simulink model "System_generator_top"  (R2025b)
settings: Solver=FixedStepAuto  StartTime=0.0  StopTime=10560000  FixedStep=1  RelTol=1e-3
InitFcn:
  | % 1. Dynamically find the exact folder where your .slx model file is saved
  | model_full_path = get_param(bdroot, 'FileName');
  | [project_dir, ~, ~] = fileparts(model_full_path);
  | input_file_path = fullfile(project_dir, 'input_video.txt');
  | 
  | % 2. Load the file directly from that project folder
  | if exist(input_file_path, 'file')
  |     fileID = fopen(input_file_path, 'r');
  |     file_contents = textscan(fileID, '%s');
  |     fclose(fileID);
  |     try
  |         raw_pixels = hex2dec(file_contents{1});
  |     catch
  |         raw_pixels = readmatrix(input_file_path);
  |         raw_pixels = raw_pixels(~isnan(raw_pixels));
  |     end
  |     total_cycles = length(raw_pixels);
  |     assignin('base', 'input_stream', [(0:total_cycles-1)', raw_pixels]);
  | 
  |     % --- THE AUTOMATION LEVEL-UP ---
  |     % Force the Simulink model stop time box to match the exact size of the video file
  |     set_param(bdroot, 'StopTime', num2str(total_cycles));
  |     fprintf('--> Automation Success: Simulink StopTime auto-set to %d to match total text pixels.\n', total_cycles);
  |     % ---------------------------------
  | else
  |     warndlg(['Warning: input_video.txt was not found in your project folder: ', project_dir]);
  | end
StopFcn:
  | try
  |     % 1. Find exactly where input_video.txt is stored
  |     input_file_full_path = which('input_video.txt');
  |     if ~isempty(input_file_full_path)
  |         [target_dir, ~, ~] = fileparts(input_file_full_path);
  |     else
  |         model_full_path = get_param(bdroot, 'FileName');
  |         [target_dir, ~, ~] = fileparts(model_full_path);
  |     end
  | 
  |     % ==========================================================
  |     % 2. STREAM EDGE PIXELS TO "output_edges.txt"
  |     % ==========================================================
  |     if exist('out', 'var') && (isprop(out, 'output_pixels') || isfield(out, 'output_pixels'))
  |         raw_output = out.output_pixels;
  |     else
  |         error('No output pixel variable found in the workspace.');
  |     end
  | 
  |     if isa(raw_output, 'Simulink.SimulationData.Signal')
  |         processed_data = raw_output.Values.Data;
  |     elseif isa(raw_output, 'timeseries')
  |         processed_data = raw_output.Data;
  |     else
  |         processed_data = raw_output;
  |     end
  | 
  |     processed_data = squeeze(double(processed_data));
  | 
  |     final_output_path = fullfile(target_dir, 'output_edges.txt');
  |     fileID = fopen(final_output_path, 'w');
  |     fprintf(fileID, '%02x\n', uint8(processed_data));
  |     fclose(fileID);
  |     fprintf('--> Automation Success: "output_edges.txt" saved.\n');
  | 
  |     % ==========================================================
  |     % 3. STREAM COORDINATES TO "box_coordinates.txt"
  |     % ==========================================================
  |     if isprop(out, 'box_min_x') || isfield(out, 'box_min_x')
  |         % Robust extraction for both Signal structures and raw timeseries classes
  |         if isa(out.box_min_x, 'Simulink.SimulationData.Signal')
  |             bx = out.box_min_x.Values.Data; Bx = out.box_max_x.Values.Data;
  |             by = out.box_min_y.Values.Data; By = out.box_max_y.Values.Data;
  |         elseif isa(out.box_min_x, 'timeseries')
  |             bx = out.box_min_x.Data; Bx = out.box_max_x.Data;
  |             by = out.box_min_y.Data; By = out.box_max_y.Data;
  |         else
  |             bx = out.box_min_x; Bx = out.box_max_x;
  |             by = out.box_min_y; By = out.box_max_y;
  |         end
  | 
  |         bx = squeeze(double(bx)); Bx = squeeze(double(Bx));
  |         by = squeeze(double(by)); By = squeeze(double(By));
  | 
  |         coords_matrix = [bx, Bx, by, By];
  | 
  |         final_coords_path = fullfile(target_dir, 'box_coordinates.txt');
  |         fileID_coords = fopen(final_coords_path, 'w');
  |         fprintf(fileID_coords, '%d %d %d %d\n', coords_matrix');
  |         fclose(fileID_coords);
  |         fprintf('--> Automation Success: "box_coordinates.txt" saved directly to your folder.\n');
  |     else
  |         warning('Coordinates missing from output structure! Check your To Workspace block names.');
  |     end
  | 
  | catch ME
  |     warning('Automation Failed: %s', ME.message);
  | end
undefined symbols (not defined in the file): gray, Subsystem, System_generator_top_exp_donot_USE, xc7z010clg400
libraries: hdlBasic x14, vmcUtilities x1
settings Model: Creator=Mayur  LastModifiedBy=Mayur

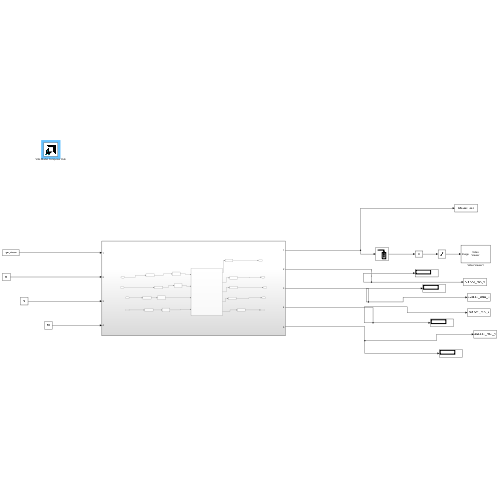
[thumbnail: Simulink's stored preview of the top-level diagram]
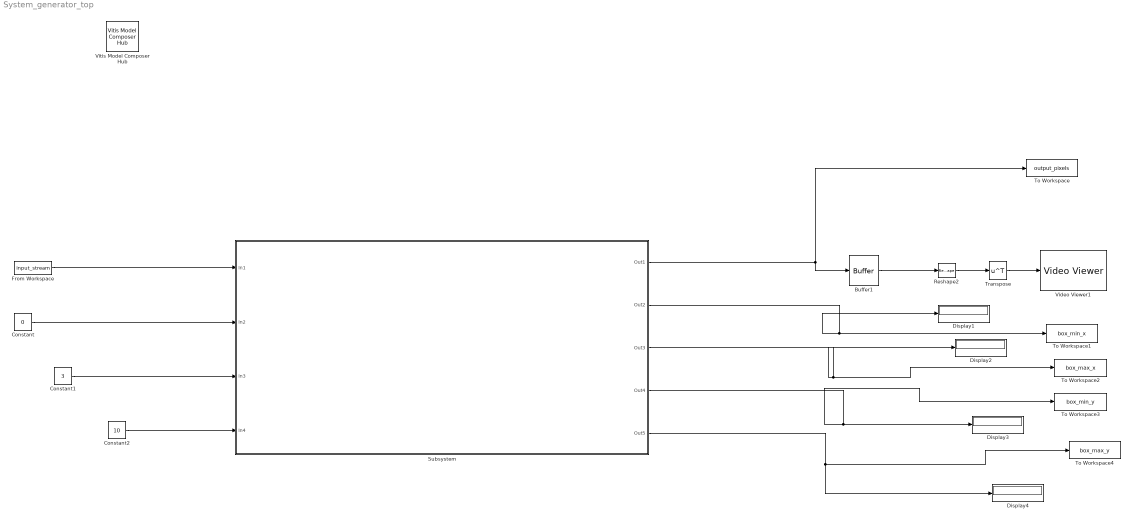
== system System_generator_top ==
  Buffer1 : Buffer  N=19200  OutputFrames=off
  Constant : Constant  Value=0  SampleTime=1  LockScale=on
  Constant1 : Constant  Value=3  SampleTime=1
  Constant2 : Constant  Value=10
  Display{1..4} (4 alike) : Display
  From Workspace : FromWorkspace  VariableName=input_stream  SampleTime=1  Interpolate=off  OutputAfterFinalValue=Holding final value
  Reshape2 : Reshape  OutputDimensionality=Customize  OutputDimensions=[160,120]
  Subsystem : Subsystem
  To Workspace : ToWorkspace  VariableName=output_pixels  SaveFormat=Timeseries  SampleTime=-1
  To Workspace1 : ToWorkspace  VariableName=box_min_x  SaveFormat=Timeseries  SampleTime=-1
  To Workspace2 : ToWorkspace  VariableName=box_max_x  SaveFormat=Timeseries  SampleTime=-1
  To Workspace3 : ToWorkspace  VariableName=box_min_y  SaveFormat=Timeseries  SampleTime=-1
  To Workspace4 : ToWorkspace  VariableName=box_max_y  SaveFormat=Timeseries  SampleTime=-1
  Transpose : Math  Operator=transpose
  Video Viewer1 : VideoViewer  colormapValue=gray(256)  FigPos=[893 880.666666666667 660 613]
  Vitis Model Composer Hub : vmcUtilities/Vitis Model Composer Hub  Tag=genX  CodeGeneration=off  SubsystemName=Subsystem  BlockHierPath=System_generator_top_exp_donot_USE/Subsystem  CompilationType=HDLCompilation  SubsystemType=HDLNode  ExportTypeV2=HDL Netlist  StartColumn=1  NumberOfColumns=1  TargetDirectory=C:/Users/Mayur/AppData/Roaming/Xilinx/Sysgen  exportDesign=on  analyzeDesign=off  validateDesignOnHw=off  ExportType=AI Engines  IpVendor=xilinx.com  IpLibrary=hls  IpVersion=1.0  IpHWLanguage=Verilog  AieCompilerOptions={}  AieSimulatorOptions={}  CreateTestbench=off  TestbenchStackSize=10  RunRtlSim=off  RunCSim=off  RunAieSim=off  AieSimTimeout=50000  RunAieSimProfiling=off  LaunchVitisAnalyzer=off  PlotOutput=off  RunX86Sim=off  X86SimTimeout=10  GenHwImage=off  GenLibadfXo=on  GenHwValidationCode=off  PlatformType=Not Specified  HwSystemType=Baremetal  HwValidationTarget=hw  ProjDevice=xc7z010clg400-1  ProjDevicePart=xc7z010clg400-1  AIEType=None  SamplePeriod=-1  ClockFrequency=200  DataPathParallelism=1  xilinxfamily=zynq  part=xc7z010  speed=-1  package=clg400  directory=./netlist\ip\Subsystem\src  testbench=off  incr_netlist=off  synthesis_tool=Vivado  clock_wrapper=Clock Enables  dbl_ovrd=According to Block Masks  dcm_input_clock_period=10  sysclk_period=10  simulink_period=1  eval_field=0  IPInfoJsonString="{\"DUTSubsystemName\":\"Subsystem\",\"HDLSubsystem\":{\"SubsystemName\":\"Subsystem\",\"IPName\":\"Subsystem\",\"IPLibrary\":\"VMC\",\"IPVendor\":\"User Company\",\"IPVersion\":\"1.0\",\"TargetDirectory\":\"C:/Users/Mayur/AppData/Roaming/Xilinx/Sysgen\",\"SubsystemDir\":\"C:/Users/Mayur/AppData/Roaming/Xilinx/Sysgen\\\\ip\\\\Subsystem\",\"FreqHz\":\"100000000\"},\"SubsystemTag\":\"HDLNode\"}"  LogFileName=C:\Users\Mayur\AppData\Roaming\Xilinx\Sysgen\model_composer.log  NThreads=4  IPConfigFile=C:\Users\Mayur\AppData\Local\Temp\vmctmp-14156349143152141850\System_generator_top_exp_donot_USE_ipconfig.json
  wires:
  Buffer1/1 -> Reshape2/1
  Reshape2/1 -> Transpose/1
  Transpose/1 -> Video Viewer1/1
  Subsystem/5(Out5) -> Display4/1, To Workspace4/1
  Subsystem/4(Out4) -> To Workspace3/1, Display3/1
  Subsystem/1(Out1) -> To Workspace/1, Buffer1/1
  Subsystem/2(Out2) -> Display1/1, To Workspace1/1
  Subsystem/3(Out3) -> To Workspace2/1, Display2/1
  From Workspace/1 -> Subsystem/1(In1)
  Constant/1 -> Subsystem/2(In2)
  Constant1/1 -> Subsystem/3(In3)
  Constant2/1 -> Subsystem/4(In4)

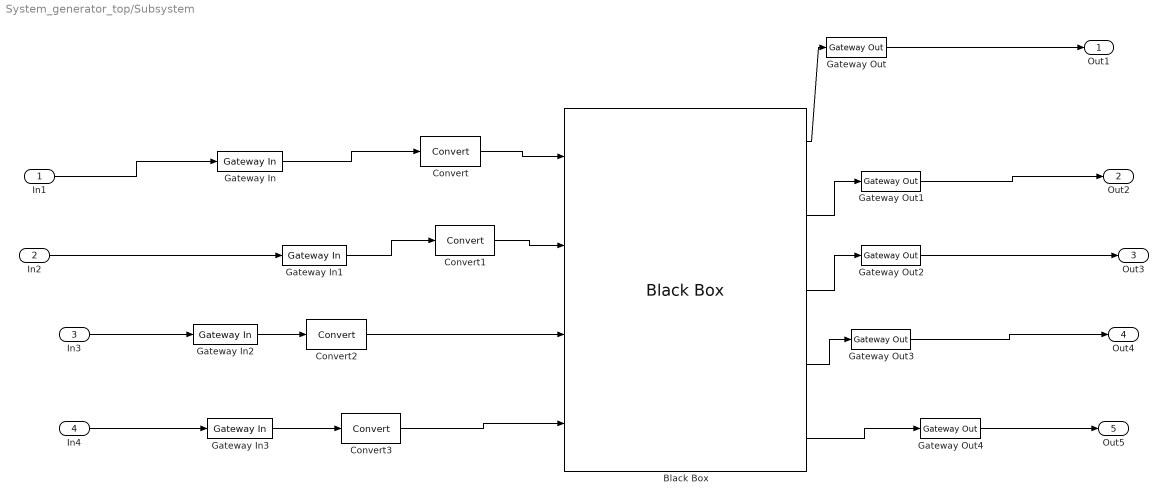
== system System_generator_top/Subsystem ==
  In1 : Inport
  In2 : Inport  Port=2
  In3 : Inport  Port=3
  In4 : Inport  Port=4
  Black Box : hdlBasic/Black Box  init_code=top_tracking_pipeline_config  sim_method=Vivado Simulator  verbose=off  XmcBlockStatus=1  maskContainerNames=group1  block_type=blackbox2  block_config=sysgen:black_box_config
  Convert : hdlBasic/Convert  gui_display_data_type=Fixed-point  arith_type=Unsigned  n_bits=8  bin_pt=0  float_type=Single  exp_bits=8  fraction_bits=24  quantization=Truncate  overflow=Wrap  en=off  latency=1  pipeline=off  XmcBlockStatus=1  maskContainerNames=group2  block_type=convert  block_config=sysgen:Convert_config  block_width=595  block_height=885
  Convert1 : hdlBasic/Convert  gui_display_data_type=Fixed-point  arith_type=Unsigned  n_bits=8  bin_pt=0  float_type=Single  exp_bits=8  fraction_bits=24  quantization=Truncate  overflow=Wrap  en=off  latency=1  pipeline=off  XmcBlockStatus=1  maskContainerNames=group2  block_type=convert  block_config=sysgen:Convert_config  block_width=595  block_height=885
  Convert2 : hdlBasic/Convert  gui_display_data_type=Fixed-point  arith_type=Unsigned  n_bits=8  bin_pt=0  float_type=Single  exp_bits=8  fraction_bits=24  quantization=Truncate  overflow=Wrap  en=off  latency=1  pipeline=off  XmcBlockStatus=1  maskContainerNames=group2  block_type=convert  block_config=sysgen:Convert_config  block_width=595  block_height=885
  Convert3 : hdlBasic/Convert  gui_display_data_type=Fixed-point  arith_type=Unsigned  n_bits=11  bin_pt=0  float_type=Single  exp_bits=8  fraction_bits=24  quantization=Truncate  overflow=Wrap  en=off  latency=1  pipeline=off  XmcBlockStatus=1  maskContainerNames=group2  block_type=convert  block_config=sysgen:Convert_config  block_width=595  block_height=885
  Gateway In : hdlBasic/Gateway In  gui_display_data_type=Fixed-point  arith_type=Signed (2's comp)  n_bits=16  bin_pt=14  preci_type=Single  exp_width=8  frac_width=24  rows=1  columns=1  quantization="Round  (unbiased: +/- Inf)"  overflow=Saturate  period=1  UseAsADC=off  ADCChannel='1'  interface=None  automatic_assignment=on  address_offset=hex2dec('00')  intf_name=''  intf_description=''  default_value=0  timing_constraint=None  locs_specified=off  LOCs={}  io_standard={}  inherit_from_input=off  hdl_port=on  XmcBlockStatus=1  maskContainerNames=group4  block_type=gatewayin  block_config=sysgen:gateway_in_config  block_width_w=590  block_height_w=620  block_width=640  block_height=850
  Gateway In1 : hdlBasic/Gateway In  gui_display_data_type=Fixed-point  arith_type=Unsigned  n_bits=8  bin_pt=0  preci_type=Single  exp_width=8  frac_width=24  rows=1  columns=1  quantization="Round  (unbiased: +/- Inf)"  overflow=Saturate  period=1  UseAsADC=off  ADCChannel='1'  interface=None  automatic_assignment=on  address_offset=hex2dec('00')  intf_name=''  intf_description=''  default_value=0  timing_constraint=None  locs_specified=off  LOCs={}  io_standard={}  inherit_from_input=off  hdl_port=on  XmcBlockStatus=1  maskContainerNames=group4  block_type=gatewayin  block_config=sysgen:gateway_in_config  block_width_w=590  block_height_w=620  block_width=640  block_height=850
  Gateway In2 : hdlBasic/Gateway In  gui_display_data_type=Fixed-point  arith_type=Unsigned  n_bits=8  bin_pt=0  preci_type=Single  exp_width=8  frac_width=24  rows=1  columns=1  quantization="Round  (unbiased: +/- Inf)"  overflow=Saturate  period=1  UseAsADC=off  ADCChannel='1'  interface=None  automatic_assignment=on  address_offset=hex2dec('00')  intf_name=''  intf_description=''  default_value=0  timing_constraint=None  locs_specified=off  LOCs={}  io_standard={}  inherit_from_input=off  hdl_port=on  XmcBlockStatus=1  maskContainerNames=group4  block_type=gatewayin  block_config=sysgen:gateway_in_config  block_width_w=590  block_height_w=620  block_width=640  block_height=850
  Gateway In3 : hdlBasic/Gateway In  gui_display_data_type=Fixed-point  arith_type=Unsigned  n_bits=11  bin_pt=0  preci_type=Single  exp_width=8  frac_width=24  rows=1  columns=1  quantization="Round  (unbiased: +/- Inf)"  overflow=Saturate  period=1  UseAsADC=off  ADCChannel='1'  interface=None  automatic_assignment=on  address_offset=hex2dec('00')  intf_name=''  intf_description=''  default_value=0  timing_constraint=None  locs_specified=off  LOCs={}  io_standard={}  inherit_from_input=off  hdl_port=on  XmcBlockStatus=1  maskContainerNames=group4  block_type=gatewayin  block_config=sysgen:gateway_in_config  block_width_w=590  block_height_w=620  block_width=640  block_height=850
  Gateway Out{,1..4} (5 alike) : hdlBasic/Gateway Out  inherit_from_input=off  bool_to_boolean=off  hdl_port=off  rows=1  columns=1  UseAsDAC=off  DACChannel='1'  interface=None  automatic_assignment=on  address_offset=hex2dec('00')  intf_name=''  intf_description=''  timing_constraint=None  locs_specified=off  LOCs={}  io_standard={}  XmcBlockStatus=1  maskContainerNames=group4  block_type=gatewayout  block_config=sysgen:gateway_out_config  block_width_w=590  block_height_w=620  block_width=620  block_height=750
  Out1 : Outport
  Out2 : Outport  Port=2
  Out3 : Outport  Port=3
  Out4 : Outport  Port=4
  Out5 : Outport  Port=5
  wires:
  Black Box/5 -> Gateway Out4/1
  Convert1/1 -> Black Box/2
  Gateway In/1 -> Convert/1
  Black Box/2 -> Gateway Out1/1
  Convert3/1 -> Black Box/4
  Gateway In2/1 -> Convert2/1
  Gateway In3/1 -> Convert3/1
  Black Box/3 -> Gateway Out2/1
  Black Box/1 -> Gateway Out/1
  Black Box/4 -> Gateway Out3/1
  Gateway Out1/1 -> Out2/1
  Gateway In1/1 -> Convert1/1
  Convert2/1 -> Black Box/3
  Convert/1 -> Black Box/1
  Gateway Out/1 -> Out1/1
  In3/1 -> Gateway In2/1
  In2/1 -> Gateway In1/1
  Gateway Out4/1 -> Out5/1
  In4/1 -> Gateway In3/1
  In1/1 -> Gateway In/1
  Gateway Out3/1 -> Out4/1
  Gateway Out2/1 -> Out3/1
